simulink model "chap7_4f2"  (Simulink 3.00)
settings: Solver=ode45  StartTime=0.0  StopTime=100  RelTol=1e-3
values from neighbouring files (symbols this model uses):
  kd = 0.20    (= 0.2)    [chap7_10.m]    (also in chap7_14.m = 0.01; chap7_15f.m = 1; chap7_2.m = 15; chap7_3f.m = 1.9688)
  ki = 0.80    (= 0.8)    [chap7_10.m]    (also in chap7_14.m = 0.01; chap7_15f.m = 10; chap7_2.m = 0; chap7_3f.m = 0.0504)
  kp = 8.0    (= 8)    [chap7_10.m]    (also in chap7_14.m = 0.1; chap7_15f.m = 50; chap7_2.m = 50; chap7_3f.m = 0.63)
libraries: simulink_extras x1

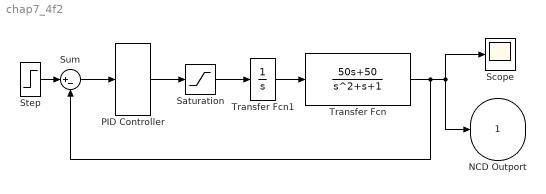
== system chap7_4f2 ==
  PID Controller : simulink_extras/Additional Linear/PID Controller  P=kp  I=ki  D=kd
  Saturation : Saturate  UpperLimit=5  LowerLimit=-5
  Scope : Scope
      settings: TimeRange=auto  YMin=-5  YMax=5  SaveToWorkspace=off  SaveName=ScopeData
  Step : Step  Time=1  Before=0  After=1  SampleTime=0
  Sum : Sum  Inputs=|+-  SaturateOnIntegerOverflow=on
  Transfer Fcn : TransferFcn  Numerator=[50 50]  Denominator=[1 1 1]
  Transfer Fcn1 : TransferFcn  Numerator=[1]  Denominator=[1 0]
  NCD Outport : Outport  Port=1  InitialOutput=0
      settings: OpenFcn=optblock
      mask Type: NCD Outport
      mask Display:
      | plot([0:10],[-.5 1.5 .6 1.3 .8 1.1 .95 1.02 .99 1 1]);
      | disp('\n\n NCD\n OutPort 1');
  wires:
  Sum/1 -> PID Controller/1
  Step/1 -> Sum/1
  Transfer Fcn/1 -> Sum/2, NCD Outport/1, Scope/1
  PID Controller/1 -> Saturation/1
  Transfer Fcn1/1 -> Transfer Fcn/1
  Saturation/1 -> Transfer Fcn1/1
